simulink model "first"  (R2014b)
settings: Solver=ode45  StartTime=0.0  StopTime=25  MaxStep=0.001  MinStep=0.0001  RelTol=1e-3
libraries: simulink x3
settings Model: Creator=Игорь  LastModifiedBy=Игорь

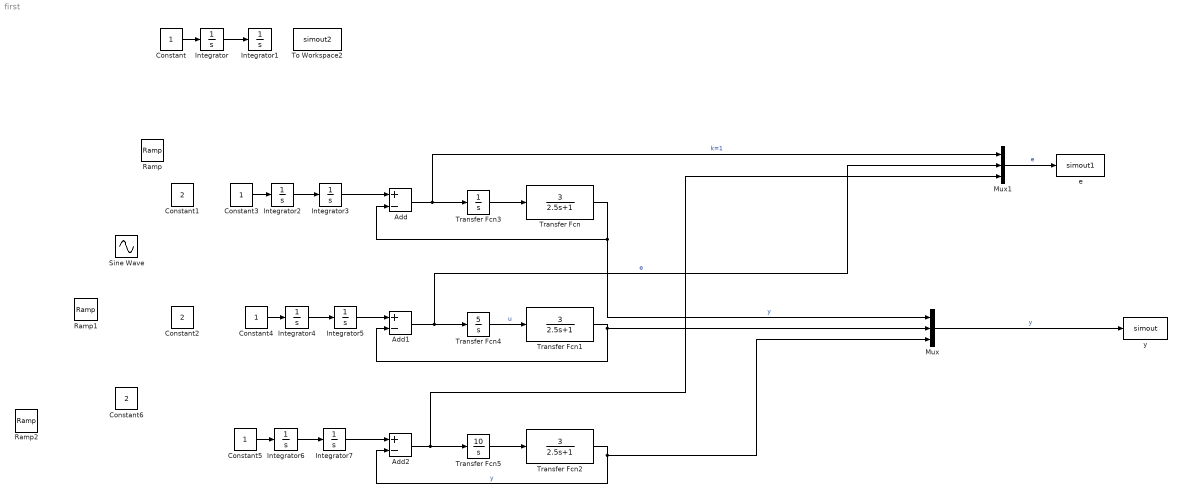
== system first ==
  Add : Sum  Inputs=+-
  Add1 : Sum  Inputs=+-
  Add2 : Sum  Inputs=+-
  Constant{,3..5} (4 alike) : Constant
  Constant1 : Constant  Value=2
  Constant2 : Constant  Value=2
  Constant6 : Constant  Value=2
  Integrator{,1..7} (8 alike) : Integrator
  Mux : Mux  Inputs=3
  Mux1 : Mux  Inputs=3
  Ramp : simulink/Sources/Ramp  slope=2  start=0  X0=0
  Ramp1 : simulink/Sources/Ramp  slope=2  start=0  X0=0
  Ramp2 : simulink/Sources/Ramp  slope=2  start=0  X0=0
  Sine Wave : Sin  SampleTime=0
  To Workspace2 : ToWorkspace  VariableName=simout2  SaveFormat=Timeseries  SampleTime=-1
  Transfer Fcn : TransferFcn  Numerator=[3]  Denominator=[2.5 1]
  Transfer Fcn1 : TransferFcn  Numerator=[3]  Denominator=[2.5 1]
  Transfer Fcn2 : TransferFcn  Numerator=[3]  Denominator=[2.5 1]
  Transfer Fcn3 : TransferFcn  Denominator=[1 0]
  Transfer Fcn4 : TransferFcn  Numerator=[5]  Denominator=[1 0]
  Transfer Fcn5 : TransferFcn  Numerator=[10]  Denominator=[1 0]
  e : ToWorkspace  VariableName=simout1  SaveFormat=Timeseries  SampleTime=-1
  y : ToWorkspace  VariableName=simout  SaveFormat=Timeseries  SampleTime=-1
  wires:
  Transfer Fcn/1 -> Mux/1, Add/2  "y"
  Add/1 -> Transfer Fcn3/1, Mux1/1  "k=1"
  Integrator/1 -> Integrator1/1
  Transfer Fcn4/1 -> Transfer Fcn1/1  "u"
  Transfer Fcn1/1 -> Add1/2, Mux/2
  Add1/1 -> Transfer Fcn4/1, Mux1/2  "e"
  Transfer Fcn2/1 -> Mux/3, Add2/2  "y"
  Add2/1 -> Transfer Fcn5/1, Mux1/3
  Mux1/1 -> e/1  "e"
  Mux/1 -> y/1  "y"
  Constant/1 -> Integrator/1
  Integrator2/1 -> Integrator3/1
  Constant3/1 -> Integrator2/1
  Integrator4/1 -> Integrator5/1
  Constant4/1 -> Integrator4/1
  Integrator6/1 -> Integrator7/1
  Constant5/1 -> Integrator6/1
  Transfer Fcn5/1 -> Transfer Fcn2/1
  Transfer Fcn3/1 -> Transfer Fcn/1
  Integrator5/1 -> Add1/1
  Integrator3/1 -> Add/1
  Integrator7/1 -> Add2/1
